simulink model "Verifica_LMI_20022026"  (R2025b)
settings: Solver=VariableStepAuto  StartTime=0.0  StopTime=20.0  RelTol=1e-3
values from neighbouring files (symbols this model uses):
  A = double(subs(A_sym, p_eq_instabile, val_instabili))    [SvolgimentoEsame.m]
  B = double(subs(B_sym, p_eq_instabile, val_instabili))    [SvolgimentoEsame.m]
  X_ref = [x_ref_val; 0; 0; 0]    [SvolgimentoEsame.m]
undefined symbols (not defined in the file or in its folder): C_tot, D_tot, K_LMI, N, X0
settings Model: Creator=salvo  LastModifiedBy=salvo

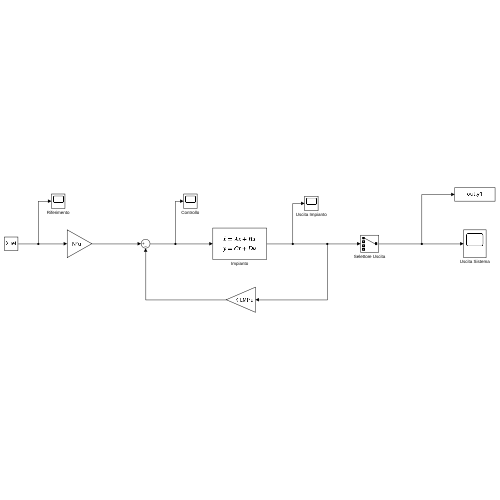
[thumbnail: Simulink's stored preview of the top-level diagram]
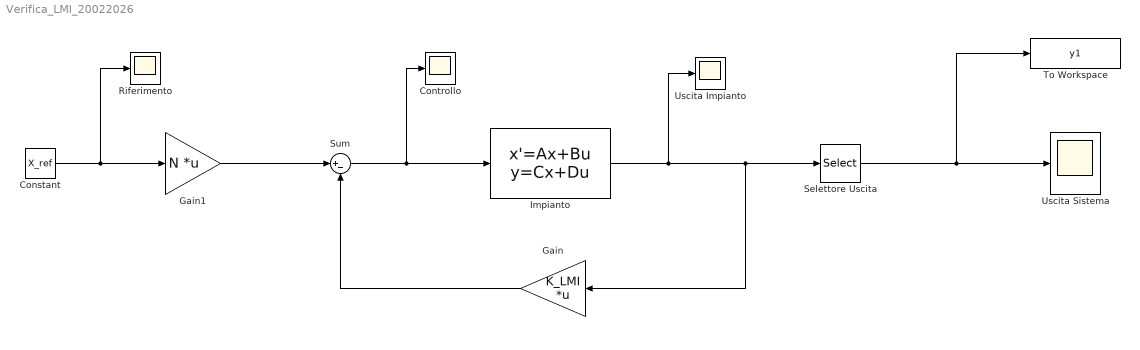
== system Verifica_LMI_20022026 ==
  Constant : Constant  Value=X_ref
  Controllo : Scope
      settings: ActiveDisplayYMinimum=-2.8975974091451882  ActiveDisplayYMaximum=9.84317113615488  DataLoggingVariableName=ScopeData2
  Gain : Gain  Gain=K_LMI  Multiplication=Matrix(K*u)
  Gain1 : Gain  Gain=N  Multiplication=Matrix(K*u)
  Impianto : StateSpace  A=A  B=B  C=C_tot  D=D_tot  InitialCondition=X0
  Riferimento : Scope
      settings: ActiveDisplayYMinimum=-0.044159750189969621  ActiveDisplayYMaximum=0.25971681231003041
  Selettore Uscita : Selector  InputPortWidth=4  IndexOptions=Index vector (dialog)  Indices=1  OutputSizes=1
  Sum : Sum  Inputs=|+-
  To Workspace : ToWorkspace  VariableName=y1  SaveFormat=Timeseries  SampleTime=-1
  Uscita Impianto : Scope
      settings: ActiveDisplayYMinimum=-1.3745276505679194  ActiveDisplayYMaximum=1.0532153296225566  DataLoggingVariableName=ScopeData3
  Uscita Sistema : Scope
      settings: ActiveDisplayYMinimum=-0.80484963453983949  ActiveDisplayYMaximum=0.93943485807882277
  wires:
  Sum/1 -> Controllo/1, Impianto/1
  Gain/1 -> Sum/2
  Impianto/1 -> Uscita Impianto/1, Gain/1, Selettore Uscita/1
  Gain1/1 -> Sum/1
  Constant/1 -> Riferimento/1, Gain1/1
  Selettore Uscita/1 -> To Workspace/1, Uscita Sistema/1
